simulink library "library"  (R2018a)
settings: Solver=ode45  StartTime=0.0  StopTime=10.0  RelTol=1e-3  EnableMultiTasking=on
undefined symbols (not defined in the file or in its folder): contr, curvature, DiscIntNeverNeededParam, k, l, pin, sysCtrl
libraries: $bdroot x16, cstblocks x1, simulink x1
(part 2 of 2)

== system library/Steering Models/Steering Model (CarMaker DSR)/a(2,2) ==
  d_rot : Inport
  d_rack : Inport  Port=2
  i : Inport  Port=3
  xi : Inport  Port=4
  Add : Sum
  Divide : Product  Inputs=*/
  Gain : Gain  Gain=-1
  Math Function : Math  Operator=square  SaturateOnIntegerOverflow=on
  Product : Product  RndMeth=Zero
  a22 : Outport
  wires:
  Gain/1 -> a22/1
  Divide/1 -> Gain/1
  d_rack/1 -> Add/2
  d_rot/1 -> Product/2
  xi/1 -> Divide/2
  i/1 -> Math Function/1
  Add/1 -> Divide/1
  Product/1 -> Add/1
  Math Function/1 -> Product/1

== system library/Steering Models/Steering Model (CarMaker DSR)/b(2,1) ==
  i : Inport
  xi : Inport  Port=2
  V : Inport  Port=3
  Math Function1 : Math  Operator=square  SaturateOnIntegerOverflow=on
  Product1 : Product  Inputs=**/  RndMeth=Zero
  b21 : Outport
  wires:
  Math Function1/1 -> Product1/1
  Product1/1 -> b21/1
  V/1 -> Product1/2
  i/1 -> Math Function1/1
  xi/1 -> Product1/3

== system library/Steering Models/Steering Model (CarMaker DSR)/b(2,2) ==
  i : Inport
  xi : Inport  Port=2
  Product1 : Product  Inputs=*/  RndMeth=Zero
  b22 : Outport
  wires:
  xi/1 -> Product1/2
  i/1 -> Product1/1
  Product1/1 -> b22/1

== system library/Steering Models/Steering Model (CarMaker DSR)/xi ==
  i : Inport
  I_rot : Inport  Port=2
  m_left : Inport  Port=3
  m_right : Inport  Port=4
  m_rack : Inport  Port=5
  Add : Sum  Inputs=++++
  Math Function : Math  Operator=square  SaturateOnIntegerOverflow=on
  Product : Product  RndMeth=Zero
  xi : Outport
  wires:
  m_rack/1 -> Add/4
  m_right/1 -> Add/3
  m_left/1 -> Add/2
  Product/1 -> Add/1
  i/1 -> Math Function/1
  Add/1 -> xi/1
  Math Function/1 -> Product/1
  I_rot/1 -> Product/2

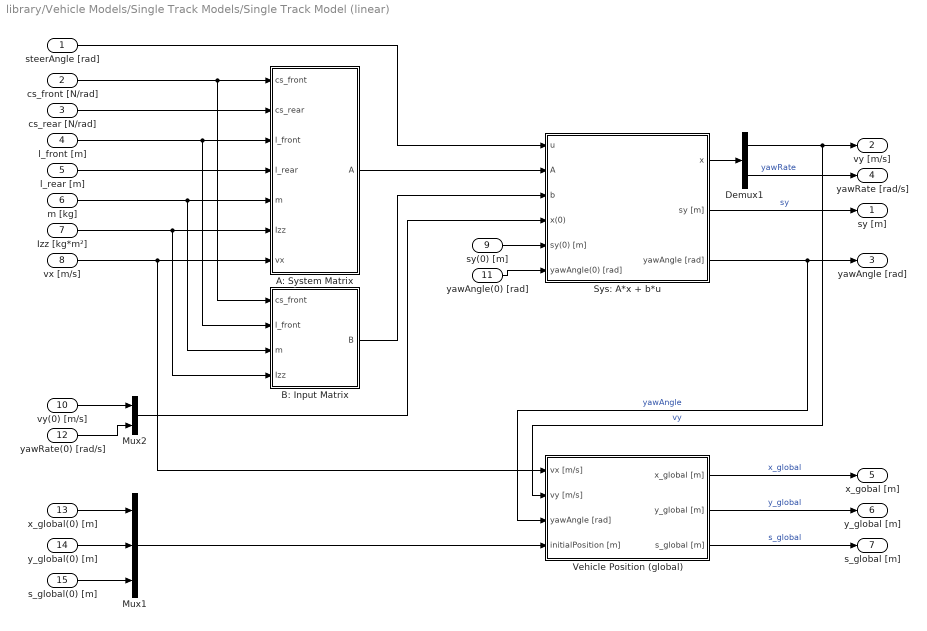
== system library/Vehicle Models/Single Track Models/Single Track Model (linear) ==
  steerAngle [rad] : Inport  OutDataTypeStr=double  PortDimensions=1
  cs_front [N/rad] : Inport  Port=2  OutDataTypeStr=double  PortDimensions=1
  cs_rear [N/rad] : Inport  Port=3  OutDataTypeStr=double  PortDimensions=1
  l_front [m] : Inport  Port=4  OutMin=0  OutDataTypeStr=double  PortDimensions=1
  l_rear [m] : Inport  Port=5  OutMin=0  OutDataTypeStr=double  PortDimensions=1
  m [kg] : Inport  Port=6  OutMin=0  OutDataTypeStr=double  PortDimensions=1
  Izz [kg*m²] : Inport  Port=7  OutMin=0  OutDataTypeStr=double  PortDimensions=1
  vx [m/s] : Inport  Port=8  OutDataTypeStr=double  PortDimensions=1
  sy(0) [m] : Inport  Port=9  OutDataTypeStr=double  PortDimensions=1
  vy(0) [m/s] : Inport  Port=10  OutDataTypeStr=double  PortDimensions=1
  yawAngle(0) [rad] : Inport  Port=11  OutDataTypeStr=double  PortDimensions=1
  yawRate(0) [rad/s] : Inport  Port=12  OutDataTypeStr=double  PortDimensions=1
  x_global(0) [m] : Inport  Port=13  OutDataTypeStr=double  PortDimensions=1
  y_global(0) [m] : Inport  Port=14  OutDataTypeStr=double  PortDimensions=1
  s_global(0) [m] : Inport  Port=15  OutDataTypeStr=double  PortDimensions=1
  A: System Matrix : Subsystem
  B: Input Matrix : Subsystem
  Demux1 : Demux  Outputs=2
  Mux1 : Mux  Inputs=3
  Mux2 : Mux  Inputs=2
  Sys: A*x + b*u : Subsystem
  Vehicle Position (global) : Subsystem
  sy [m] : Outport  OutDataTypeStr=double  PortDimensions=1
  vy [m/s] : Outport  Port=2  OutDataTypeStr=double  PortDimensions=1
  yawAngle [rad] : Outport  Port=3  OutDataTypeStr=double  PortDimensions=1
  yawRate [rad/s] : Outport  Port=4  OutDataTypeStr=double  PortDimensions=1
  x_gobal [m] : Outport  Port=5  OutDataTypeStr=double  PortDimensions=1
  y_global [m] : Outport  Port=6  OutDataTypeStr=double  PortDimensions=1
  s_global [m] : Outport  Port=7  OutDataTypeStr=double  PortDimensions=1
  wires:
  steerAngle [rad]/1 -> Sys: A*x + b*u/1(u)
  cs_front [N/rad]/1 -> A: System Matrix/1(cs_front), B: Input Matrix/1(cs_front)
  cs_rear [N/rad]/1 -> A: System Matrix/2(cs_rear)
  l_front [m]/1 -> A: System Matrix/3(l_front), B: Input Matrix/2(l_front)
  l_rear [m]/1 -> A: System Matrix/4(l_rear)
  m [kg]/1 -> A: System Matrix/5(m), B: Input Matrix/3(m)
  Izz [kg*m²]/1 -> A: System Matrix/6(Izz), B: Input Matrix/4(Izz)
  vx [m/s]/1 -> A: System Matrix/7(vx), Vehicle Position (global)/1(vx [m/s])
  Sys: A*x + b*u/2(sy [m]) -> sy [m]/1  "sy"
  Sys: A*x + b*u/3(yawAngle [rad]) -> yawAngle [rad]/1, Vehicle Position (global)/3(yawAngle [rad])  "yawAngle"
  Demux1/2 -> yawRate [rad/s]/1  "yawRate"
  Vehicle Position (global)/1(x_global [m]) -> x_gobal [m]/1  "x_global"
  Vehicle Position (global)/2(y_global [m]) -> y_global [m]/1  "y_global"
  Vehicle Position (global)/3(s_global [m]) -> s_global [m]/1  "s_global"
  vy(0) [m/s]/1 -> Mux2/1
  yawRate(0) [rad/s]/1 -> Mux2/2
  x_global(0) [m]/1 -> Mux1/1
  y_global(0) [m]/1 -> Mux1/2
  s_global(0) [m]/1 -> Mux1/3
  Mux1/1 -> Vehicle Position (global)/4(initialPosition [m])
  A: System Matrix/1(A) -> Sys: A*x + b*u/2(A)
  B: Input Matrix/1(B) -> Sys: A*x + b*u/3(b)
  Mux2/1 -> Sys: A*x + b*u/4(x(0))
  sy(0) [m]/1 -> Sys: A*x + b*u/5(sy(0) [m])
  yawAngle(0) [rad]/1 -> Sys: A*x + b*u/6(yawAngle(0) [rad])
  Sys: A*x + b*u/1(x) -> Demux1/1
  Demux1/1 -> vy [m/s]/1, Vehicle Position (global)/2(vy [m/s])  "vy"

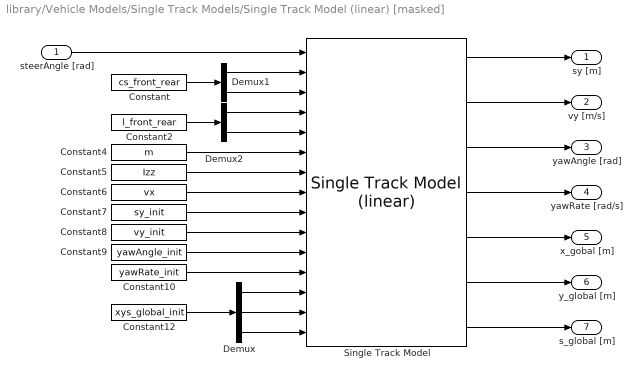
== system library/Vehicle Models/Single Track Models/Single Track Model (linear) [masked] ==
  steerAngle [rad] : Inport
  Constant : Constant  Value=cs_front_rear
  Constant10 : Constant  Value=yawRate_init
  Constant12 : Constant  Value=xys_global_init
  Constant2 : Constant  Value=l_front_rear
  Constant4 : Constant  Value=m
  Constant5 : Constant  Value=Izz
  Constant6 : Constant  Value=vx
  Constant7 : Constant  Value=sy_init
  Constant8 : Constant  Value=vy_init
  Constant9 : Constant  Value=yawAngle_init
  Demux : Demux  Outputs=3
  Demux1 : Demux  Outputs=2
  Demux2 : Demux  Outputs=2
  Single Track Model : $bdroot/Vehicle Models/Single Track Models/Single Track Model (linear)
  sy [m] : Outport
  vy [m/s] : Outport  Port=2
  yawAngle [rad] : Outport  Port=3
  yawRate [rad/s] : Outport  Port=4
  x_gobal [m] : Outport  Port=5
  y_global [m] : Outport  Port=6
  s_global [m] : Outport  Port=7
  wires:
  steerAngle [rad]/1 -> Single Track Model/1
  Constant4/1 -> Single Track Model/6
  Constant5/1 -> Single Track Model/7
  Constant6/1 -> Single Track Model/8
  Single Track Model/1 -> sy [m]/1
  Single Track Model/2 -> vy [m/s]/1
  Single Track Model/3 -> yawAngle [rad]/1
  Single Track Model/4 -> yawRate [rad/s]/1
  Single Track Model/5 -> x_gobal [m]/1
  Single Track Model/6 -> y_global [m]/1
  Single Track Model/7 -> s_global [m]/1
  Constant7/1 -> Single Track Model/9
  Constant8/1 -> Single Track Model/10
  Constant9/1 -> Single Track Model/11
  Constant10/1 -> Single Track Model/12
  Constant12/1 -> Demux/1
  Demux/1 -> Single Track Model/13
  Demux/2 -> Single Track Model/14
  Demux/3 -> Single Track Model/15
  Demux1/1 -> Single Track Model/2
  Demux1/2 -> Single Track Model/3
  Constant/1 -> Demux1/1
  Demux2/1 -> Single Track Model/4
  Demux2/2 -> Single Track Model/5
  Constant2/1 -> Demux2/1

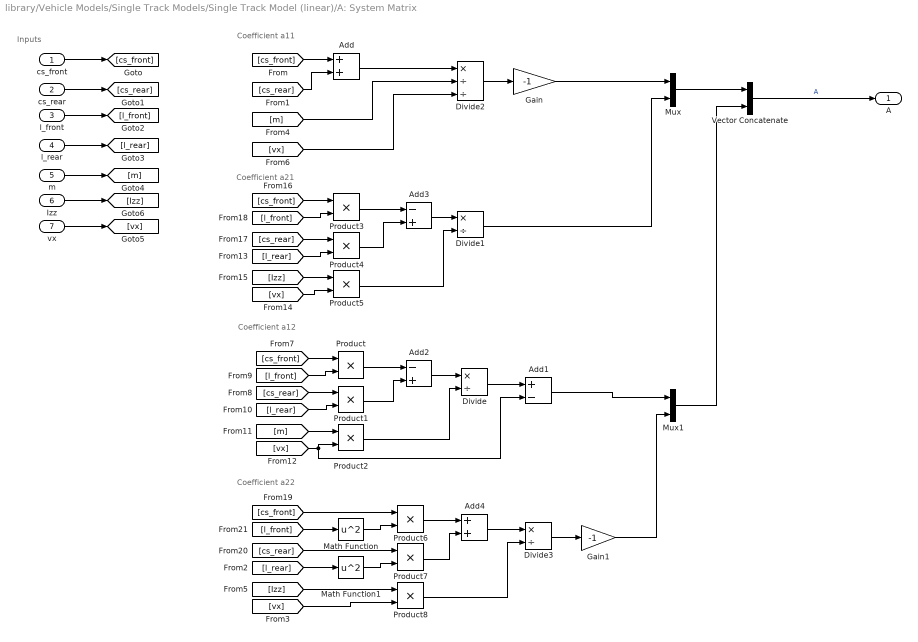
== system library/Vehicle Models/Single Track Models/Single Track Model (linear)/A: System Matrix ==
  note: Inputs
  note: Coefficient a21
  note: Coefficient a12
  note: Coefficient a11
  note: Coefficient a22
  cs_front : Inport
  cs_rear : Inport  Port=2
  l_front : Inport  Port=3
  l_rear : Inport  Port=4
  m : Inport  Port=5
  Izz : Inport  Port=6
  vx : Inport  Port=7
  Add : Sum
  Add1 : Sum  Inputs=+-
  Add2 : Sum  Inputs=-+
  Add3 : Sum  Inputs=-+
  Add4 : Sum
  Divide : Product  Inputs=*/
  Divide1 : Product  Inputs=*/
  Divide2 : Product  Inputs=*//
  Divide3 : Product  Inputs=*/
  Gain : Gain  Gain=-1
  Gain1 : Gain  Gain=-1
  Math Function : Math  Operator=square  SaturateOnIntegerOverflow=on
  Math Function1 : Math  Operator=square  SaturateOnIntegerOverflow=on
  Mux : Mux  Inputs=2
  Mux1 : Mux  Inputs=2
  Product{,1..8} (9 alike) : Product  RndMeth=Zero
  Vector Concatenate : Concatenate  Mode=Multidimensional array  ConcatenateDimension=2
  A : Outport
  wires:
  Mux/1 -> Vector Concatenate/1
  Mux1/1 -> Vector Concatenate/2
  Vector Concatenate/1 -> A/1  "A"
  Divide1/1 -> Mux/2
  Gain/1 -> Mux/1
  [cs_front] -> Add/1
  [vx] -> Divide2/3
  Divide2/1 -> Gain/1
  [m] -> Divide2/2
  [cs_rear] -> Add/2
  Add/1 -> Divide2/1
  cs_front/1 -> [cs_front]
  cs_rear/1 -> [cs_rear]
  l_front/1 -> [l_front]
  vx/1 -> [vx]
  l_rear/1 -> [l_rear]
  m/1 -> [m]
  Izz/1 -> [Izz]
  Product2/1 -> Divide/2
  Product1/1 -> Add2/2
  Product/1 -> Add2/1
  Add2/1 -> Divide/1
  [vx] -> Add1/2, Product2/2
  [m] -> Product2/1
  Add1/1 -> Mux1/1
  [l_front] -> Product/2
  [cs_rear] -> Product1/1
  Divide/1 -> Add1/1
  [l_rear] -> Product1/2
  [cs_front] -> Product/1
  [Izz] -> Product5/1
  [l_front] -> Product3/2
  Product3/1 -> Add3/1
  Add3/1 -> Divide1/1
  Product5/1 -> Divide1/2
  [cs_front] -> Product3/1
  [vx] -> Product5/2
  [l_rear] -> Product4/2
  Product4/1 -> Add3/2
  [cs_rear] -> Product4/1
  [vx] -> Product8/2
  [l_rear] -> Math Function1/1
  Math Function/1 -> Product6/2
  Product8/1 -> Divide3/2
  Math Function1/1 -> Product7/2
  Divide3/1 -> Gain1/1
  Product7/1 -> Add4/2
  [Izz] -> Product8/1
  [l_front] -> Math Function/1
  Product6/1 -> Add4/1
  [cs_rear] -> Product7/1
  Gain1/1 -> Mux1/2
  Add4/1 -> Divide3/1
  [cs_front] -> Product6/1

== system library/Vehicle Models/Single Track Models/Single Track Model (linear)/B: Input Matrix ==
  cs_front : Inport
  l_front : Inport  Port=2
  m : Inport  Port=3
  Izz : Inport  Port=4
  Divide : Product  Inputs=*/
  Divide1 : Product  Inputs=**/
  Mux : Mux  Inputs=2
  B : Outport
  wires:
  cs_front/1 -> Divide/1, Divide1/1
  m/1 -> Divide/2
  Izz/1 -> Divide1/3
  l_front/1 -> Divide1/2
  Divide/1 -> Mux/1
  Divide1/1 -> Mux/2
  Mux/1 -> B/1

== system library/Vehicle Models/Single Track Models/Single Track Model (linear)/Sys: A*x + b*u ==
  u : Inport
  A : Inport  Port=2
  b : Inport  Port=3
  x(0) : Inport  Port=4
  sy(0) [m] : Inport  Port=5  OutDataTypeStr=double  PortDimensions=1
  yawAngle(0) [rad] : Inport  Port=6  OutDataTypeStr=double  PortDimensions=1
  A*x : Product  Multiplication=Matrix(*)  RndMeth=Zero
  Demux1 : Demux  Outputs=2
  Integrator1 : Integrator  InitialConditionSource=external
  Integrator2 : Integrator  InitialConditionSource=external
  Mux2 : Mux  Inputs=2
  Sum : Sum  Inputs=++|
  b*u : Product  Multiplication=Matrix(*)  RndMeth=Zero
  x : Outport  OutDataTypeStr=double  PortDimensions=2
  sy [m] : Outport  Port=2  OutDataTypeStr=double  PortDimensions=1
  yawAngle [rad] : Outport  Port=3  OutDataTypeStr=double  PortDimensions=1
  wires:
  Sum/1 -> Integrator1/1
  Integrator1/1 -> A*x/2, Integrator2/1, x/1
  A/1 -> A*x/1
  x(0)/1 -> Integrator1/2
  b/1 -> b*u/1
  u/1 -> b*u/2
  A*x/1 -> Sum/2
  b*u/1 -> Sum/1
  sy(0) [m]/1 -> Mux2/1
  yawAngle(0) [rad]/1 -> Mux2/2
  Mux2/1 -> Integrator2/2
  Integrator2/1 -> Demux1/1
  Demux1/1 -> sy [m]/1
  Demux1/2 -> yawAngle [rad]/1

== system library/Vehicle Models/Single Track Models/Single Track Model (linear)/Vehicle Position (global) ==
  vx [m/s] : Inport
  vy [m/s] : Inport  Port=2
  yawAngle [rad] : Inport  Port=3
  initialPosition [m] : Inport  Port=4
  Demux : Demux  Outputs=3
  Fcn1 : Fcn  Expr=u(1)*cos(u(3)) - u(2)*sin(u(3))
  Fcn2 : Fcn  Expr=u(1)*sin(u(3)) + u(2)*cos(u(3))
  Fcn3 : Fcn  Expr=sqrt( u(1)^2 + u(2)^2 )
  Integrator1 : Integrator  InitialConditionSource=external
  Integrator2 : Integrator  InitialConditionSource=external
  Integrator3 : Integrator  InitialConditionSource=external
  Mux : Mux  Inputs=3
  x_global [m] : Outport
  y_global [m] : Outport  Port=2
  s_global [m] : Outport  Port=3
  wires:
  Integrator2/1 -> y_global [m]/1
  yawAngle [rad]/1 -> Mux/3
  vy [m/s]/1 -> Mux/2
  vx [m/s]/1 -> Mux/1
  Integrator1/1 -> x_global [m]/1
  Fcn2/1 -> Integrator2/1
  Fcn1/1 -> Integrator1/1
  Fcn3/1 -> Integrator3/1
  Integrator3/1 -> s_global [m]/1
  Mux/1 -> Fcn2/1, Fcn1/1, Fcn3/1
  initialPosition [m]/1 -> Demux/1
  Demux/1 -> Integrator1/2
  Demux/2 -> Integrator2/2
  Demux/3 -> Integrator3/2

== matlab function library/Lane Tracking/Lane Tracking Sensor/MATLAB Function ==
  data: LAD input; isValid_LAD input; lateralOff_LAD input; angularDev_LAD input; roadCurvat_LAD input; poly_lateralOff_LAD output; poly_angularDev_LAD output; poly_roadCurvat_LAD output; poly_domain_LAD output
function [...
 poly_lateralOff_LAD,...
 poly_angularDev_LAD,...
 poly_roadCurvat_LAD,...
 poly_domain_LAD] = polyFitLaneSensor(...
 LAD,...
 isValid_LAD,...
 lateralOff_LAD,...
 angularDev_LAD,...
 roadCurvat_LAD)
%#codegen


%%% number of valid measurements specify maximum degree of polynomial
np_max = sum(isValid_LAD) - 1;

if any(~isValid_LAD)
	1;
end%if

%%% init outputs
% choose polynomial degree/fixed output length
np = 3;
poly_lateralOff_LAD	= zeros(1,np+1);
poly_angularDev_LAD	= zeros(1,np+1);
poly_roadCurvat_LAD	= zeros(1,np+1);

%%% fit polynomial coefficients
n = min(np,np_max);
LAD_valid = LAD(isValid_LAD);
poly_latOff	= polyfit(LAD_valid,lateralOff_LAD(isValid_LAD),n);
poly_angDev	= polyfit(LAD_valid,angularDev_LAD(isValid_LAD),n);
poly_rdCurv	= polyfit(LAD_valid,roadCurvat_LAD(isValid_LAD),n);

%%% add coefficients to output
poly_lateralOff_LAD(np-n+1:np+1) = poly_latOff;
poly_angularDev_LAD(np-n+1:np+1) = poly_angDev;
poly_roadCurvat_LAD(np-n+1:np+1) = poly_rdCurv;

poly_domain_LAD = [min(LAD_valid);max(LAD_valid)];

end%fcn
